simulink model "topology_comparison_cur"  (R2024b)
settings: Solver=ode23tb  StartTime=0.0  StopTime=0.15  MaxStep=1e-5  MinStep=1e-8  RelTol=1e-4
InitFcn:
  | sw_freq=60e3;
  | 
  | meas_delay=0.1;
  | 
  | V_high=80;
  | V_low=70;
  | 
  | L_ind=300e-6;
  | L_res=20e-3;
  | MOS_Ron=10e-3;
  | MOS_Vfw=1.2;
  | DIO_Vfw=1;
  | DIO_Ron=1e-3;
  | TRC_Res=5e-3;
  | 
  | buck_p=0.01;
  | buck_i=2;
  | 
  | inter_bdc_p=0.01;
  | inter_bdc_i=2;
  | 
  | asym_bdc_p=0.01;
  | asym_bdc_i=2;
values from neighbouring files (symbols this model uses):
  i_low_ref = 0.25    [compare_conv_curr.m]
  mode = 0    [compare_conv_curr.m]
libraries: spsGroundLib x33, spsSeriesRLCBranchLib x33, spsMosfetLib x18, spsDCVoltageSourceLib x14, spsMeanLib x10, slpidlib x10, spsMultimeterLib x6, spsVoltageMeasurementLib x4, spsDiodeLib x2, spsCurrentMeasurementLib x2, sps_lib x1
(part 1 of 2)
settings Model: SimulationMode=rapid-accelerator  Creator=adamo  LastModifiedBy=adamo
settings DebuggingCC: MaskedZcDiagnostic=none  IgnoredZcDiagnostic=none
settings HardwareCC: ProdHWDeviceType=AMD->x86-64 (Windows64)
settings RTWCC: BuildConfiguration=Faster Runs  CheckMdlBeforeBuild=Error
settings GRTTargetCC: OptimizeReductions=on
settings SimscapeCC: SimscapeCompileComponentReuse=on  SimscapeCompileArtifactsDiskCache=on

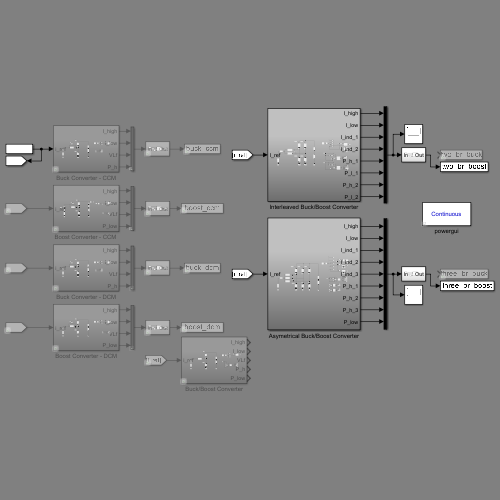
[thumbnail: Simulink's stored preview of the top-level diagram]
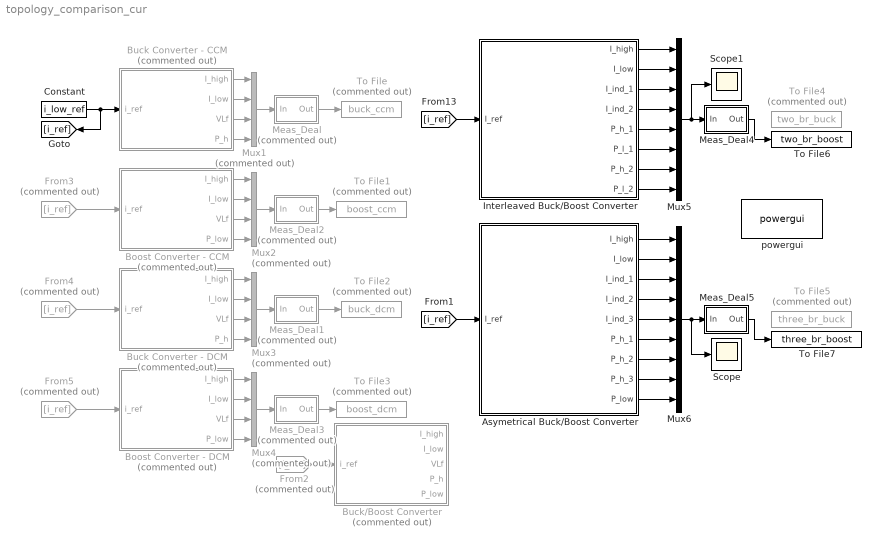
== system topology_comparison_cur ==
  Asymetrical Buck/Boost Converter : Subsystem
  "Boost Converter - CCM " : Subsystem  Commented=on
  Boost Converter - DCM : Subsystem  Commented=on
  Buck Converter - CCM : Subsystem  Commented=on
  Buck Converter - DCM : Subsystem  Commented=on
  Buck/Boost Converter : Subsystem  Commented=on
  Constant : Constant  Value=i_low_ref
  From{2..5} (4 alike) : From  Commented=on  GotoTag=i_ref
  Interleaved Buck/Boost Converter : Subsystem
  Meas_Deal : Subsystem  Commented=on
  Meas_Deal1 : Subsystem  Commented=on
  Meas_Deal2 : Subsystem  Commented=on
  Meas_Deal3 : Subsystem  Commented=on
  Meas_Deal4 : Subsystem
  Meas_Deal5 : Subsystem
  Mux{1..4} (4 alike) : Mux  Commented=on
  Mux5 : Mux  Inputs=8
  Mux6 : Mux  Inputs=9
  Scope : Scope
  Scope1 : Scope
  To File : ToFile  Commented=on  Filename=buck_ccm
  To File1 : ToFile  Commented=on  Filename=boost_ccm
  To File2 : ToFile  Commented=on  Filename=buck_dcm
  To File3 : ToFile  Commented=on  Filename=boost_dcm
  To File4 : ToFile  Commented=on  Filename=two_br_buck
  To File5 : ToFile  Commented=on  Filename=three_br_buck
  To File6 : ToFile  Filename=two_br_boost
  To File7 : ToFile  Filename=three_br_boost
  powergui : sps_lib/powergui  Priority=1  SimulationMode=Continuous  SampleTime=50e-6  frequency=60  Iterations=50  frequencyindice=0  Pbase=100e6  ErrMax=1e-4  UnitsV=kV  UnitsW=MW  buscounter=0  FunctionMessages=off  echomessages=off  EnableUseOfTLC=off  CurrentSourceSwitches=off  DisableSnubberDevices=on  DisableRonSwitches=off  DisableVfSwitches=off  DisplayEquations=off  AutomaticDiscreteSolvers=off  SolverType=Tustin/Backward Euler (TBE)  Interpol=off  ExternalGateDelay=off  methode=on  Ts=100  x0status=blocks  SPID=on  SwTol=0  HookPort=off  NonlinearTolerance=1e-4  nMaxIteration=100  ContinueOnMaxIteration=off  RestoreLinks=warning  ResistiveCurrentMeasurement=off  Frange=[0:2:500]  Ylog=off  Xlog=on  ShowGrid=off  save=off  variable=ZData  structure=0  ZoomFFT=off  StartTime=0.0  cycles=1  DisplayStyle=1  fundamental=60  FreqAxis=off  MaxFrequency=1000  frequencyindicesteady=1  RmsSteady=1  display=off
  wires:
  Buck Converter - CCM/2(I_low) -> Mux1/2
  Constant/1 -> [i_ref], Buck Converter - CCM/1(i_ref)
  [i_ref] -> Interleaved Buck/Boost Converter/1(I_ref)
  [i_ref] -> Asymetrical Buck/Boost Converter/1(I_ref)
  Buck Converter - CCM/3(VLf) -> Mux1/3
  Buck Converter - CCM/4(P_h) -> Mux1/4
  Meas_Deal/1(Out) -> To File/1
  From3/1 -> "Boost Converter - CCM "/1(i_ref)
  Meas_Deal2/1(Out) -> To File1/1
  "Boost Converter - CCM "/4(P_low) -> Mux2/4
  "Boost Converter - CCM "/3(VLf) -> Mux2/3
  "Boost Converter - CCM "/1(I_high) -> Mux2/1
  "Boost Converter - CCM "/2(I_low) -> Mux2/2
  Mux2/1 -> Meas_Deal2/1(In)
  From2/1 -> Buck/Boost Converter/1(i_ref)
  Buck Converter - CCM/1(I_high) -> Mux1/1
  Meas_Deal1/1(Out) -> To File2/1
  Meas_Deal3/1(Out) -> To File3/1
  Boost Converter - DCM/3(VLf) -> Mux4/3
  Buck Converter - DCM/3(VLf) -> Mux3/3
  Mux3/1 -> Meas_Deal1/1(In)
  Buck Converter - DCM/2(I_low) -> Mux3/2
  Buck Converter - DCM/4(P_h) -> Mux3/4
  Mux4/1 -> Meas_Deal3/1(In)
  From4/1 -> Buck Converter - DCM/1(i_ref)
  Boost Converter - DCM/2(I_low) -> Mux4/2
  Boost Converter - DCM/4(P_low) -> Mux4/4
  Buck Converter - DCM/1(I_high) -> Mux3/1
  From5/1 -> Boost Converter - DCM/1(i_ref)
  Boost Converter - DCM/1(I_high) -> Mux4/1
  Mux1/1 -> Meas_Deal/1(In)
  Interleaved Buck/Boost Converter/1(I_high) -> Mux5/1
  Interleaved Buck/Boost Converter/2(I_low) -> Mux5/2
  Interleaved Buck/Boost Converter/3(I_ind_1) -> Mux5/3
  Interleaved Buck/Boost Converter/4(I_ind_2) -> Mux5/4
  Interleaved Buck/Boost Converter/5(P_h_1) -> Mux5/5
  Interleaved Buck/Boost Converter/6(P_l_1) -> Mux5/6
  Interleaved Buck/Boost Converter/7(P_h_2) -> Mux5/7
  Interleaved Buck/Boost Converter/8(P_l_2) -> Mux5/8
  Meas_Deal4/1(Out) -> To File6/1
  Mux5/1 -> Scope1/1, Meas_Deal4/1(In)
  Asymetrical Buck/Boost Converter/1(I_high) -> Mux6/1
  Asymetrical Buck/Boost Converter/2(I_low) -> Mux6/2
  Asymetrical Buck/Boost Converter/3(I_ind_1) -> Mux6/3
  Asymetrical Buck/Boost Converter/4(I_ind_2) -> Mux6/4
  Asymetrical Buck/Boost Converter/5(I_ind_3) -> Mux6/5
  Asymetrical Buck/Boost Converter/6(P_h_1) -> Mux6/6
  Asymetrical Buck/Boost Converter/7(P_h_2) -> Mux6/7
  Asymetrical Buck/Boost Converter/8(P_h_3) -> Mux6/8
  Asymetrical Buck/Boost Converter/9(P_low) -> Mux6/9
  Mux6/1 -> Scope/1, Meas_Deal5/1(In)
  Meas_Deal5/1(Out) -> To File7/1

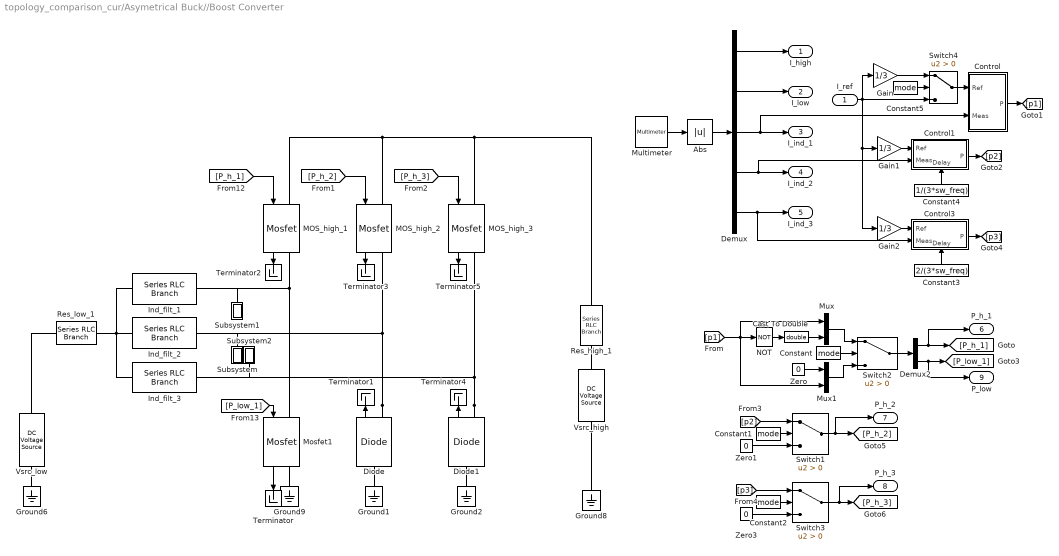
== system topology_comparison_cur/Asymetrical Buck//Boost Converter ==
  I_ref : Inport
  Abs : Abs  SaturateOnIntegerOverflow=off
  Cast To Double : DataTypeConversion  OutDataTypeStr=double  SaturateOnIntegerOverflow=off  RndMeth=Floor
  Constant{,1..2,5} (4 alike) : Constant  Value=mode
  Constant3 : Constant  Value=2/(3*sw_freq)
  Constant4 : Constant  Value=1/(3*sw_freq)
  Control : Subsystem
  Control1 : Subsystem
      settings: PortSchema="{\"entries\":[{\"content\":{\"sides\":[{\"content\":{\"connectorIds\":[\"In1\",\"In2\"]},\"type\":\"ConnectorPlacement.EquallySpacedRectSide\",\"uuid\":\"44975c06-6cb3-4b92-aa2e-c11b859d13e4\"},{\"content\":{\"connectorIds\":[\"Out1\"],\"side\":\"RIGHT\"},\"type\":\"ConnectorPlacement.EquallySpacedRectSide\",\"uuid\":\"ebdc9065-5b19-4aa7-8841-916fd82a5d31\"},{\"content\":{\"side\":\"TOP\"},\"type\":\"ConnectorPlacement.EquallySpacedRectSide\",\"uuid\":\"027925ea-888b-4bcf-b8a4-44694d0e275e\"},{\"content\":{\"connectorIds\":[\"In3\"],\"side\":\"BOTTOM\"},\"type\":\"ConnectorPlacement.EquallySpacedRectSide\",\"uuid\":\"415fb0af-dd9a-4309-9118-76332ed11379\"}]},\"type\":\"ConnectorPlacement.EquallySpacedConnector\",\"uuid\":\"3cd19595-535e-42c3-a0e6-40045bedee28\"}],\"packageUris\":[\"http://schema.mathworks.com/mf0/Connector/R2020b\"],\"version\":\"1.0\"}"
  Control3 : Subsystem
      settings: PortSchema="{\"entries\":[{\"content\":{\"sides\":[{\"content\":{\"connectorIds\":[\"In1\",\"In2\"]},\"type\":\"ConnectorPlacement.EquallySpacedRectSide\",\"uuid\":\"44975c06-6cb3-4b92-aa2e-c11b859d13e4\"},{\"content\":{\"connectorIds\":[\"Out1\"],\"side\":\"RIGHT\"},\"type\":\"ConnectorPlacement.EquallySpacedRectSide\",\"uuid\":\"ebdc9065-5b19-4aa7-8841-916fd82a5d31\"},{\"content\":{\"side\":\"TOP\"},\"type\":\"ConnectorPlacement.EquallySpacedRectSide\",\"uuid\":\"027925ea-888b-4bcf-b8a4-44694d0e275e\"},{\"content\":{\"connectorIds\":[\"In3\"],\"side\":\"BOTTOM\"},\"type\":\"ConnectorPlacement.EquallySpacedRectSide\",\"uuid\":\"9488b47a-c58c-42e9-bacd-7bb9f563b775\"}]},\"type\":\"ConnectorPlacement.EquallySpacedConnector\",\"uuid\":\"3cd19595-535e-42c3-a0e6-40045bedee28\"}],\"packageUris\":[\"http://schema.mathworks.com/mf0/Connector/R2020b\"],\"version\":\"1.0\"}"
  Demux : Demux  Outputs=5
  Demux2 : Demux  Outputs=2
  Diode : spsDiodeLib/Diode  Ron=0.001  Lon=0  Vf=0.8  IC=0  UseSnubber=0  Rs=500  Cs=250e-9  Measurements=on
  Diode1 : spsDiodeLib/Diode  Ron=0.001  Lon=0  Vf=0.8  IC=0  UseSnubber=0  Rs=500  Cs=250e-9  Measurements=on
  Gain : Gain  Gain=1/3
  Gain1 : Gain  Gain=1/3
  Gain2 : Gain  Gain=1/3
  Ground{1..2,6,8..9} (5 alike) : spsGroundLib/Ground  LConnTagsString=a
  Ind_filt_1 : spsSeriesRLCBranchLib/Series RLC Branch  LConnTagsString=__new0  RConnTagsString=__new0  BranchType=RL  Resistance=L_res  Inductance=L_ind*7  SetiL0=off  InitialCurrent=10  Capacitance=1e-6  Setx0=off  InitialVoltage=0  Measurements=Branch current
  Ind_filt_2 : spsSeriesRLCBranchLib/Series RLC Branch  LConnTagsString=__new0  RConnTagsString=__new0  BranchType=RL  Resistance=L_res  Inductance=L_ind*7  SetiL0=off  InitialCurrent=10  Capacitance=1e-6  Setx0=off  InitialVoltage=0  Measurements=Branch current
  Ind_filt_3 : spsSeriesRLCBranchLib/Series RLC Branch  LConnTagsString=__new0  RConnTagsString=__new0  BranchType=RL  Resistance=L_res  Inductance=L_ind*7  SetiL0=off  InitialCurrent=10  Capacitance=1e-6  Setx0=off  InitialVoltage=0  Measurements=Branch current
  MOS_high_1 : spsMosfetLib/Mosfet  Ron=MOS_Ron  Lon=0  Rd=DIO_Ron  Vfd=MOS_Vfw  IC=0  Rs=1e5  Cs=inf  Measurements=on
  MOS_high_2 : spsMosfetLib/Mosfet  Ron=MOS_Ron  Lon=0  Rd=DIO_Ron  Vfd=MOS_Vfw  IC=0  Rs=1e5  Cs=inf  Measurements=on
  MOS_high_3 : spsMosfetLib/Mosfet  Ron=MOS_Ron  Lon=0  Rd=DIO_Ron  Vfd=MOS_Vfw  IC=0  Rs=1e5  Cs=inf  Measurements=on
  Mosfet1 : spsMosfetLib/Mosfet  Ron=0.1  Lon=0  Rd=0.01  Vfd=0  IC=0  Rs=1e5  Cs=inf  Measurements=on
  Multimeter : spsMultimeterLib/Multimeter  L=9  sel=[4 5 1 2 3]  yselected={}  Gain=[1 1 1 1 1]  OutputType=Complex  PlotAtSimulationStop=off  PhasorSimulation=off
  Mux : Mux  Inputs=2
  Mux1 : Mux  Inputs=2
  NOT : Logic  Operator=NOT  IconShape=distinctive  AllPortsSameDT=off  OutDataTypeStr=boolean
  Res_high_1 : spsSeriesRLCBranchLib/Series RLC Branch  LConnTagsString=__new0  RConnTagsString=__new0  BranchType=R  Resistance=TRC_Res  Inductance=1e-3  SetiL0=off  InitialCurrent=0  Capacitance=1e-6  Setx0=off  InitialVoltage=0  Measurements=Branch current
  Res_low_1 : spsSeriesRLCBranchLib/Series RLC Branch  LConnTagsString=__new0  RConnTagsString=__new0  BranchType=R  Resistance=TRC_Res  Inductance=1e-3  SetiL0=off  InitialCurrent=0  Capacitance=1e-6  Setx0=off  InitialVoltage=0  Measurements=Branch current
  Subsystem : Subsystem
      settings: PortSchema="{\"entries\":[{\"content\":{\"sides\":[{\"content\":{},\"type\":\"ConnectorPlacement.EquallySpacedRectSide\",\"uuid\":\"333a472d-5660-403e-9749-9e5a485a4e51\"},{\"content\":{\"side\":\"RIGHT\"},\"type\":\"ConnectorPlacement.EquallySpacedRectSide\",\"uuid\":\"46e3a3df-9b43-4056-bf49-6d97e0ff375e\"},{\"content\":{\"connectorIds\":[\"LConn1\"],\"side\":\"TOP\"},\"type\":\"ConnectorPlacement.EquallySpacedRectSide\",\"uuid\":\"a9be43b9-3284-437d-b483-2a714199e3a2\"}]},\"type\":\"ConnectorPlacement.EquallySpacedConnector\",\"uuid\":\"6030dd83-63ea-4a67-9f73-95d000b3af89\"}],\"packageUris\":[\"http://schema.mathworks.com/mf0/Connector/R2020b\"],\"version\":\"1.0\"}"
  Subsystem1 : Subsystem
      settings: PortSchema="{\"entries\":[{\"content\":{\"sides\":[{\"content\":{},\"type\":\"ConnectorPlacement.EquallySpacedRectSide\",\"uuid\":\"333a472d-5660-403e-9749-9e5a485a4e51\"},{\"content\":{\"side\":\"RIGHT\"},\"type\":\"ConnectorPlacement.EquallySpacedRectSide\",\"uuid\":\"46e3a3df-9b43-4056-bf49-6d97e0ff375e\"},{\"content\":{\"connectorIds\":[\"LConn1\"],\"side\":\"TOP\"},\"type\":\"ConnectorPlacement.EquallySpacedRectSide\",\"uuid\":\"a9be43b9-3284-437d-b483-2a714199e3a2\"}]},\"type\":\"ConnectorPlacement.EquallySpacedConnector\",\"uuid\":\"6030dd83-63ea-4a67-9f73-95d000b3af89\"}],\"packageUris\":[\"http://schema.mathworks.com/mf0/Connector/R2020b\"],\"version\":\"1.0\"}"
  Subsystem2 : Subsystem
      settings: PortSchema="{\"entries\":[{\"content\":{\"sides\":[{\"content\":{},\"type\":\"ConnectorPlacement.EquallySpacedRectSide\",\"uuid\":\"333a472d-5660-403e-9749-9e5a485a4e51\"},{\"content\":{\"side\":\"RIGHT\"},\"type\":\"ConnectorPlacement.EquallySpacedRectSide\",\"uuid\":\"46e3a3df-9b43-4056-bf49-6d97e0ff375e\"},{\"content\":{\"connectorIds\":[\"LConn1\"],\"side\":\"TOP\"},\"type\":\"ConnectorPlacement.EquallySpacedRectSide\",\"uuid\":\"a9be43b9-3284-437d-b483-2a714199e3a2\"}]},\"type\":\"ConnectorPlacement.EquallySpacedConnector\",\"uuid\":\"6030dd83-63ea-4a67-9f73-95d000b3af89\"}],\"packageUris\":[\"http://schema.mathworks.com/mf0/Connector/R2020b\"],\"version\":\"1.0\"}"
  Switch{1..4} (4 alike) : Switch  Criteria=u2 > Threshold  SaturateOnIntegerOverflow=off  InputSameDT=off
  Terminator{,1..5} (6 alike) : Terminator
  Vsrc_high : spsDCVoltageSourceLib/DC Voltage Source  Amplitude=V_high  Measurements=None
  Vsrc_low : spsDCVoltageSourceLib/DC Voltage Source  Amplitude=V_low  Measurements=None
  Zero : Constant  Value=0  OutDataTypeStr=Inherit: Inherit via back propagation
  Zero1 : Constant  Value=0  OutDataTypeStr=Inherit: Inherit via back propagation
  Zero3 : Constant  Value=0  OutDataTypeStr=Inherit: Inherit via back propagation
  I_high : Outport
  I_low : Outport  Port=2
  I_ind_1 : Outport  Port=3
  I_ind_2 : Outport  Port=4
  I_ind_3 : Outport  Port=5
  P_h_1 : Outport  Port=6
  P_h_2 : Outport  Port=7
  P_h_3 : Outport  Port=8
  P_low : Outport  Port=9
  wires:
  [P_h_1] -> MOS_high_1/1
  MOS_high_1/1 -> Terminator2/1
  Mosfet1/1 -> Terminator/1
  [P_low_1] -> Mosfet1/1
  Diode/1 -> Terminator1/1
  MOS_high_2/1 -> Terminator3/1
  Diode1/1 -> Terminator4/1
  MOS_high_3/1 -> Terminator5/1
  [P_h_3] -> MOS_high_3/1
  Multimeter/1 -> Abs/1
  Switch2/1 -> Demux2/1
  Mux/1 -> Switch2/1
  Demux2/2 -> P_low/1, [P_low_1]
  Demux2/1 -> P_h_1/1, [P_h_1]
  Constant/1 -> Switch2/2
  I_ref/1 -> Gain/1, Switch4/3, Gain2/1, Gain1/1
  [P_h_2] -> MOS_high_2/1
  Demux/5 -> Control3/2(Meas), I_ind_3/1
  Demux/3 -> Control/2(Meas), I_ind_1/1
  Mux1/1 -> Switch2/3
  Cast To Double/1 -> Mux/2
  Demux/2 -> I_low/1
  Demux/1 -> I_high/1
  Abs/1 -> Demux/1
  Switch4/1 -> Control/1(Ref)
  Control/1(P) -> [p1]
  Control1/1(P) -> [p2]
  Gain1/1 -> Control1/1(Ref)
  Demux/4 -> Control1/2(Meas), I_ind_2/1
  Gain2/1 -> Control3/1(Ref)
  Control3/1(P) -> [p3]
  Switch3/1 -> P_h_3/1, [P_h_3]
  Switch1/1 -> P_h_2/1, [P_h_2]
  Constant1/1 -> Switch1/2
  [p2] -> Switch1/1
  Zero1/1 -> Switch1/3
  Constant2/1 -> Switch3/2
  [p3] -> Switch3/1
  Zero3/1 -> Switch3/3
  Constant4/1 -> Control1/3(Delay)
  Constant3/1 -> Control3/3(Delay)
  NOT/1 -> Cast To Double/1
  [p1] -> NOT/1, Mux/1, Mux1/2
  Constant5/1 -> Switch4/2
  Gain/1 -> Switch4/1
  Zero/1 -> Mux1/1
  connections:
  Diode/RConn1 -- Ind_filt_2/LConn1 -- Subsystem/LConn1 -- MOS_high_2/RConn1
  MOS_high_1/RConn1 -- Ind_filt_1/LConn1 -- Subsystem1/LConn1 -- Mosfet1/LConn1
  Ground8/LConn1 -- Vsrc_high/LConn1
  Mosfet1/RConn1 -- Ground9/LConn1
  Ground6/LConn1 -- Vsrc_low/LConn1
  Diode/LConn1 -- Ground1/LConn1
  Diode1/RConn1 -- Ind_filt_3/LConn1 -- Subsystem2/LConn1 -- MOS_high_3/RConn1
  Diode1/LConn1 -- Ground2/LConn1
  Res_low_1/RConn1 -- Vsrc_low/RConn1
  Res_high_1/LConn1 -- Vsrc_high/RConn1
  Ind_filt_2/RConn1 -- Res_low_1/LConn1 -- Ind_filt_3/RConn1 -- Ind_filt_1/RConn1
  Res_high_1/RConn1 -- MOS_high_1/LConn1 -- MOS_high_2/LConn1 -- MOS_high_3/LConn1

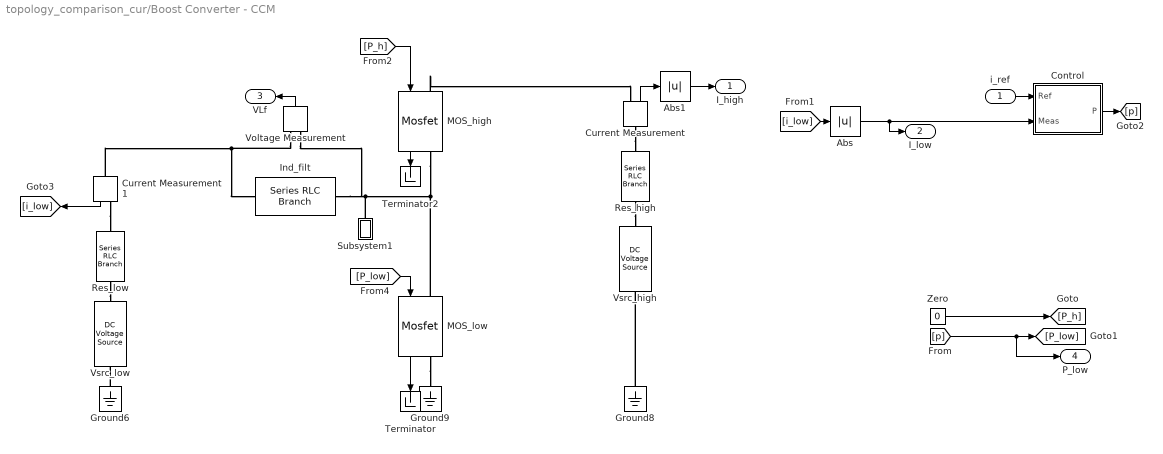
== system topology_comparison_cur/Boost Converter - CCM  ==
  i_ref : Inport
  Abs : Abs  SaturateOnIntegerOverflow=off
  Abs1 : Abs  SaturateOnIntegerOverflow=off
  Control : Subsystem
  Current Measurement : spsCurrentMeasurementLib/Current Measurement  PhasorSimulation=off  OutputType=Complex  PSBequivalent=0
  Current Measurement1 : spsCurrentMeasurementLib/Current Measurement  PhasorSimulation=off  OutputType=Complex  PSBequivalent=0
  Ground6 : spsGroundLib/Ground  LConnTagsString=a
  Ground8 : spsGroundLib/Ground  LConnTagsString=a
  Ground9 : spsGroundLib/Ground  LConnTagsString=a
  Ind_filt : spsSeriesRLCBranchLib/Series RLC Branch  LConnTagsString=__new0  RConnTagsString=__new0  BranchType=RL  Resistance=L_res  Inductance=L_ind  SetiL0=off  InitialCurrent=20  Capacitance=1e-6  Setx0=off  InitialVoltage=0  Measurements=None
  MOS_high : spsMosfetLib/Mosfet  Ron=MOS_Ron  Lon=0  Rd=DIO_Ron  Vfd=MOS_Vfw  IC=0  Rs=1e5  Cs=inf  Measurements=on
  MOS_low : spsMosfetLib/Mosfet  Ron=MOS_Ron  Lon=0  Rd=DIO_Ron  Vfd=MOS_Vfw  IC=0  Rs=1e5  Cs=inf  Measurements=on
  Res_high : spsSeriesRLCBranchLib/Series RLC Branch  LConnTagsString=__new0  RConnTagsString=__new0  BranchType=R  Resistance=TRC_Res  Inductance=1e-3  SetiL0=off  InitialCurrent=0  Capacitance=1e-6  Setx0=off  InitialVoltage=0  Measurements=None
  Res_low : spsSeriesRLCBranchLib/Series RLC Branch  LConnTagsString=__new0  RConnTagsString=__new0  BranchType=R  Resistance=TRC_Res  Inductance=1e-3  SetiL0=off  InitialCurrent=0  Capacitance=1e-6  Setx0=off  InitialVoltage=0  Measurements=None
  Subsystem1 : Subsystem
      settings: PortSchema="{\"entries\":[{\"content\":{\"sides\":[{\"content\":{},\"type\":\"ConnectorPlacement.EquallySpacedRectSide\",\"uuid\":\"333a472d-5660-403e-9749-9e5a485a4e51\"},{\"content\":{\"side\":\"RIGHT\"},\"type\":\"ConnectorPlacement.EquallySpacedRectSide\",\"uuid\":\"46e3a3df-9b43-4056-bf49-6d97e0ff375e\"},{\"content\":{\"connectorIds\":[\"LConn1\"],\"side\":\"TOP\"},\"type\":\"ConnectorPlacement.EquallySpacedRectSide\",\"uuid\":\"a9be43b9-3284-437d-b483-2a714199e3a2\"}]},\"type\":\"ConnectorPlacement.EquallySpacedConnector\",\"uuid\":\"6030dd83-63ea-4a67-9f73-95d000b3af89\"}],\"packageUris\":[\"http://schema.mathworks.com/mf0/Connector/R2020b\"],\"version\":\"1.0\"}"
  Terminator : Terminator
  Terminator2 : Terminator
  Voltage Measurement : spsVoltageMeasurementLib/Voltage Measurement  PhasorSimulation=off  OutputType=Complex  PSBequivalent=0
  Vsrc_high : spsDCVoltageSourceLib/DC Voltage Source  Amplitude=V_high  Measurements=None
  Vsrc_low : spsDCVoltageSourceLib/DC Voltage Source  Amplitude=V_low  Measurements=None
  Zero : Constant  Value=0  OutDataTypeStr=Inherit: Inherit via back propagation
  I_high : Outport
  I_low : Outport  Port=2
  VLf : Outport  Port=3
  P_low : Outport  Port=4
  wires:
  MOS_low/1 -> Terminator/1
  MOS_high/1 -> Terminator2/1
  [P_h] -> MOS_high/1
  [P_low] -> MOS_low/1
  Abs/1 -> I_low/1, Control/2(Meas)
  Zero/1 -> [P_h]
  i_ref/1 -> Control/1(Ref)
  [p] -> P_low/1, [P_low]
  Control/1(P) -> [p]
  Voltage Measurement/1 -> VLf/1
  Current Measurement/1 -> Abs1/1
  Current Measurement1/1 -> [i_low]
  [i_low] -> Abs/1
  Abs1/1 -> I_high/1
  connections:
  MOS_high/LConn1 -- Current Measurement/RConn1
  MOS_low/RConn1 -- Ground9/LConn1
  MOS_high/RConn1 -- Subsystem1/LConn1 -- Voltage Measurement/LConn1 -- Ind_filt/LConn1 -- MOS_low/LConn1
  Ground8/LConn1 -- Vsrc_high/LConn1
  Ground6/LConn1 -- Vsrc_low/LConn1
  Voltage Measurement/LConn2 -- Ind_filt/RConn1 -- Current Measurement1/LConn1
  Res_high/LConn1 -- Vsrc_high/RConn1
  Res_low/RConn1 -- Vsrc_low/RConn1
  Current Measurement/LConn1 -- Res_high/RConn1
  Current Measurement1/RConn1 -- Res_low/LConn1

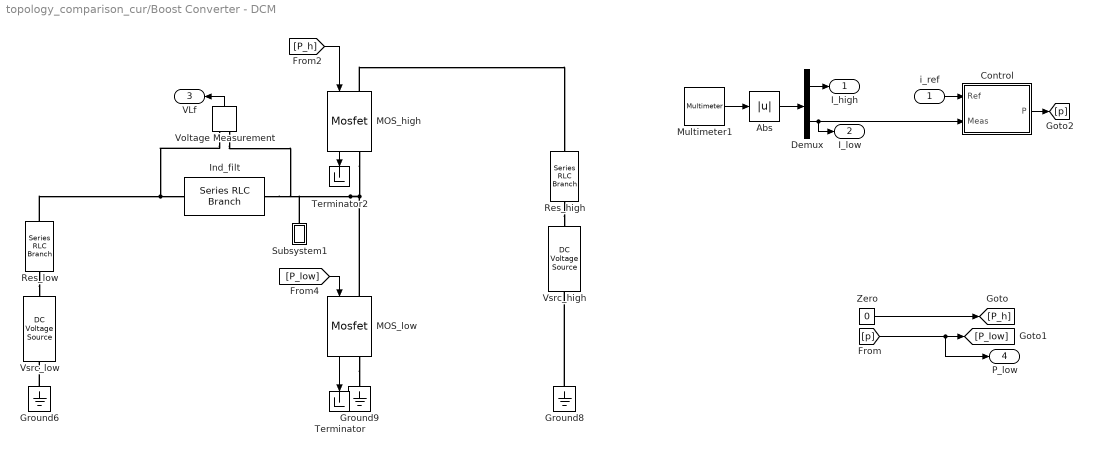
== system topology_comparison_cur/Boost Converter - DCM ==
  i_ref : Inport
  Abs : Abs  SaturateOnIntegerOverflow=off
  Control : Subsystem
  Demux : Demux  Outputs=2
  Ground6 : spsGroundLib/Ground  LConnTagsString=a
  Ground8 : spsGroundLib/Ground  LConnTagsString=a
  Ground9 : spsGroundLib/Ground  LConnTagsString=a
  Ind_filt : spsSeriesRLCBranchLib/Series RLC Branch  LConnTagsString=__new0  RConnTagsString=__new0  BranchType=RL  Resistance=L_res  Inductance=L_ind/30  SetiL0=off  InitialCurrent=20  Capacitance=1e-6  Setx0=off  InitialVoltage=0  Measurements=None
  MOS_high : spsMosfetLib/Mosfet  Ron=MOS_Ron  Lon=0  Rd=DIO_Ron  Vfd=MOS_Vfw  IC=0  Rs=1e5  Cs=inf  Measurements=on
  MOS_low : spsMosfetLib/Mosfet  Ron=MOS_Ron  Lon=0  Rd=DIO_Ron  Vfd=MOS_Vfw  IC=0  Rs=1e5  Cs=inf  Measurements=on
  Multimeter1 : spsMultimeterLib/Multimeter  L=6  sel=[1 2]  yselected={}  Gain=[1 1]  OutputType=Complex  PlotAtSimulationStop=off  PhasorSimulation=off
  Res_high : spsSeriesRLCBranchLib/Series RLC Branch  LConnTagsString=__new0  RConnTagsString=__new0  BranchType=R  Resistance=TRC_Res  Inductance=1e-3  SetiL0=off  InitialCurrent=0  Capacitance=1e-6  Setx0=off  InitialVoltage=0  Measurements=Branch current
  Res_low : spsSeriesRLCBranchLib/Series RLC Branch  LConnTagsString=__new0  RConnTagsString=__new0  BranchType=R  Resistance=TRC_Res  Inductance=1e-3  SetiL0=off  InitialCurrent=0  Capacitance=1e-6  Setx0=off  InitialVoltage=0  Measurements=Branch current
  Subsystem1 : Subsystem
      settings: PortSchema="{\"entries\":[{\"content\":{\"sides\":[{\"content\":{},\"type\":\"ConnectorPlacement.EquallySpacedRectSide\",\"uuid\":\"333a472d-5660-403e-9749-9e5a485a4e51\"},{\"content\":{\"side\":\"RIGHT\"},\"type\":\"ConnectorPlacement.EquallySpacedRectSide\",\"uuid\":\"46e3a3df-9b43-4056-bf49-6d97e0ff375e\"},{\"content\":{\"connectorIds\":[\"LConn1\"],\"side\":\"TOP\"},\"type\":\"ConnectorPlacement.EquallySpacedRectSide\",\"uuid\":\"a9be43b9-3284-437d-b483-2a714199e3a2\"}]},\"type\":\"ConnectorPlacement.EquallySpacedConnector\",\"uuid\":\"6030dd83-63ea-4a67-9f73-95d000b3af89\"}],\"packageUris\":[\"http://schema.mathworks.com/mf0/Connector/R2020b\"],\"version\":\"1.0\"}"
  Terminator : Terminator
  Terminator2 : Terminator
  Voltage Measurement : spsVoltageMeasurementLib/Voltage Measurement  PhasorSimulation=off  OutputType=Complex  PSBequivalent=0
  Vsrc_high : spsDCVoltageSourceLib/DC Voltage Source  Amplitude=V_high  Measurements=None
  Vsrc_low : spsDCVoltageSourceLib/DC Voltage Source  Amplitude=V_low  Measurements=None
  Zero : Constant  Value=0  OutDataTypeStr=Inherit: Inherit via back propagation
  I_high : Outport
  I_low : Outport  Port=2
  VLf : Outport  Port=3
  P_low : Outport  Port=4
  wires:
  MOS_low/1 -> Terminator/1
  MOS_high/1 -> Terminator2/1
  [P_h] -> MOS_high/1
  [P_low] -> MOS_low/1
  Demux/1 -> I_high/1
  Demux/2 -> I_low/1, Control/2(Meas)
  Zero/1 -> [P_h]
  i_ref/1 -> Control/1(Ref)
  Multimeter1/1 -> Abs/1
  [p] -> P_low/1, [P_low]
  Abs/1 -> Demux/1
  Control/1(P) -> [p]
  Voltage Measurement/1 -> VLf/1
  connections:
  MOS_high/LConn1 -- Res_high/RConn1
  MOS_low/RConn1 -- Ground9/LConn1
  MOS_high/RConn1 -- MOS_low/LConn1 -- Voltage Measurement/LConn1 -- Ind_filt/LConn1 -- Subsystem1/LConn1
  Ground8/LConn1 -- Vsrc_high/LConn1
  Ground6/LConn1 -- Vsrc_low/LConn1
  Res_low/LConn1 -- Ind_filt/RConn1 -- Voltage Measurement/LConn2
  Res_high/LConn1 -- Vsrc_high/RConn1
  Res_low/RConn1 -- Vsrc_low/RConn1

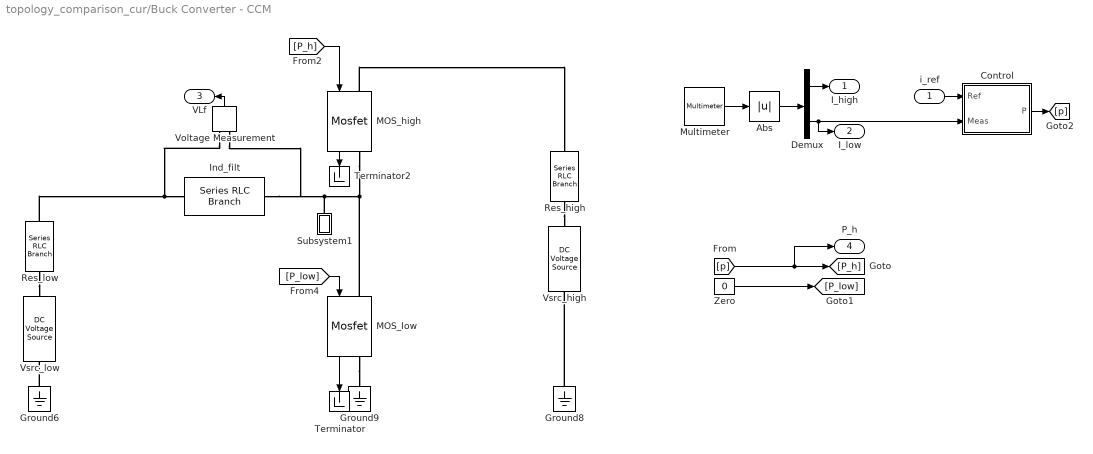
== system topology_comparison_cur/Buck Converter - CCM ==
  i_ref : Inport
  Abs : Abs  SaturateOnIntegerOverflow=off
  Control : Subsystem
  Demux : Demux  Outputs=2
  Ground6 : spsGroundLib/Ground  LConnTagsString=a
  Ground8 : spsGroundLib/Ground  LConnTagsString=a
  Ground9 : spsGroundLib/Ground  LConnTagsString=a
  Ind_filt : spsSeriesRLCBranchLib/Series RLC Branch  LConnTagsString=__new0  RConnTagsString=__new0  BranchType=RL  Resistance=L_res  Inductance=L_ind  SetiL0=off  InitialCurrent=20  Capacitance=1e-6  Setx0=off  InitialVoltage=0  Measurements=None
  MOS_high : spsMosfetLib/Mosfet  Ron=MOS_Ron  Lon=0  Rd=DIO_Ron  Vfd=MOS_Vfw  IC=0  Rs=1e5  Cs=inf  Measurements=on
  MOS_low : spsMosfetLib/Mosfet  Ron=MOS_Ron  Lon=0  Rd=DIO_Ron  Vfd=MOS_Vfw  IC=0  Rs=1e5  Cs=inf  Measurements=on
  Multimeter : spsMultimeterLib/Multimeter  L=6  sel=[3 4]  yselected={}  Gain=[1 1]  OutputType=Complex  PlotAtSimulationStop=off  PhasorSimulation=off
  Res_high : spsSeriesRLCBranchLib/Series RLC Branch  LConnTagsString=__new0  RConnTagsString=__new0  BranchType=R  Resistance=TRC_Res  Inductance=1e-3  SetiL0=off  InitialCurrent=0  Capacitance=1e-6  Setx0=off  InitialVoltage=0  Measurements=Branch current
  Res_low : spsSeriesRLCBranchLib/Series RLC Branch  LConnTagsString=__new0  RConnTagsString=__new0  BranchType=R  Resistance=TRC_Res  Inductance=1e-3  SetiL0=off  InitialCurrent=0  Capacitance=1e-6  Setx0=off  InitialVoltage=0  Measurements=Branch current
  Subsystem1 : Subsystem
      settings: PortSchema="{\"entries\":[{\"content\":{\"sides\":[{\"content\":{},\"type\":\"ConnectorPlacement.EquallySpacedRectSide\",\"uuid\":\"333a472d-5660-403e-9749-9e5a485a4e51\"},{\"content\":{\"side\":\"RIGHT\"},\"type\":\"ConnectorPlacement.EquallySpacedRectSide\",\"uuid\":\"46e3a3df-9b43-4056-bf49-6d97e0ff375e\"},{\"content\":{\"connectorIds\":[\"LConn1\"],\"side\":\"TOP\"},\"type\":\"ConnectorPlacement.EquallySpacedRectSide\",\"uuid\":\"a9be43b9-3284-437d-b483-2a714199e3a2\"}]},\"type\":\"ConnectorPlacement.EquallySpacedConnector\",\"uuid\":\"6030dd83-63ea-4a67-9f73-95d000b3af89\"}],\"packageUris\":[\"http://schema.mathworks.com/mf0/Connector/R2020b\"],\"version\":\"1.0\"}"
  Terminator : Terminator
  Terminator2 : Terminator
  Voltage Measurement : spsVoltageMeasurementLib/Voltage Measurement  PhasorSimulation=off  OutputType=Complex  PSBequivalent=0
  Vsrc_high : spsDCVoltageSourceLib/DC Voltage Source  Amplitude=V_high  Measurements=None
  Vsrc_low : spsDCVoltageSourceLib/DC Voltage Source  Amplitude=V_low  Measurements=None
  Zero : Constant  Value=0  OutDataTypeStr=Inherit: Inherit via back propagation
  I_high : Outport
  I_low : Outport  Port=2
  VLf : Outport  Port=3
  P_h : Outport  Port=4
  wires:
  MOS_low/1 -> Terminator/1
  MOS_high/1 -> Terminator2/1
  [P_h] -> MOS_high/1
  [P_low] -> MOS_low/1
  Demux/1 -> I_high/1
  Demux/2 -> I_low/1, Control/2(Meas)
  [p] -> P_h/1, [P_h]
  i_ref/1 -> Control/1(Ref)
  Multimeter/1 -> Abs/1
  Zero/1 -> [P_low]
  Abs/1 -> Demux/1
  Control/1(P) -> [p]
  Voltage Measurement/1 -> VLf/1
  connections:
  MOS_high/LConn1 -- Res_high/RConn1
  MOS_low/RConn1 -- Ground9/LConn1
  MOS_high/RConn1 -- Subsystem1/LConn1 -- Voltage Measurement/LConn1 -- Ind_filt/LConn1 -- MOS_low/LConn1
  Ground8/LConn1 -- Vsrc_high/LConn1
  Ground6/LConn1 -- Vsrc_low/LConn1
  Res_low/LConn1 -- Voltage Measurement/LConn2 -- Ind_filt/RConn1
  Res_high/LConn1 -- Vsrc_high/RConn1
  Res_low/RConn1 -- Vsrc_low/RConn1

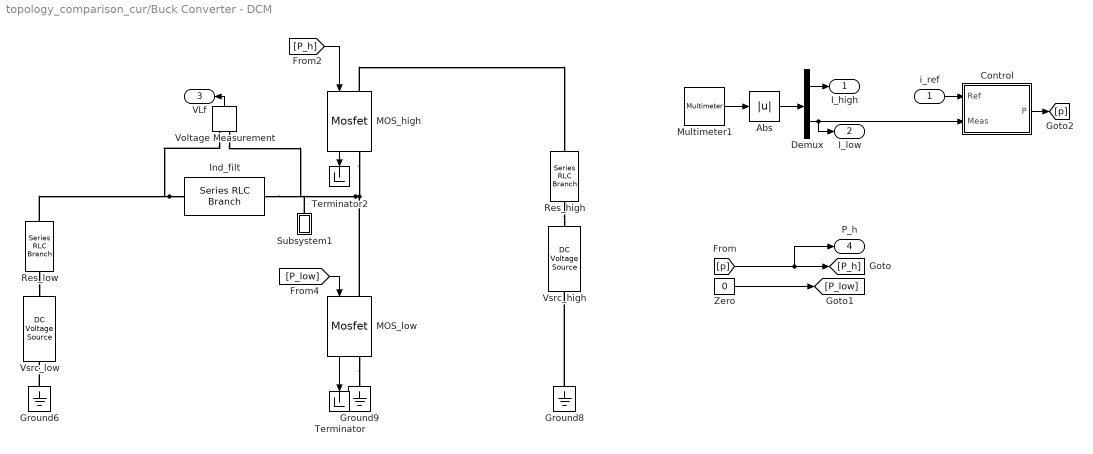
== system topology_comparison_cur/Buck Converter - DCM ==
  i_ref : Inport
  Abs : Abs  SaturateOnIntegerOverflow=off
  Control : Subsystem
  Demux : Demux  Outputs=2
  Ground6 : spsGroundLib/Ground  LConnTagsString=a
  Ground8 : spsGroundLib/Ground  LConnTagsString=a
  Ground9 : spsGroundLib/Ground  LConnTagsString=a
  Ind_filt : spsSeriesRLCBranchLib/Series RLC Branch  LConnTagsString=__new0  RConnTagsString=__new0  BranchType=RL  Resistance=L_res  Inductance=L_ind/30  SetiL0=off  InitialCurrent=20  Capacitance=1e-6  Setx0=off  InitialVoltage=0  Measurements=None
  MOS_high : spsMosfetLib/Mosfet  Ron=MOS_Ron  Lon=0  Rd=DIO_Ron  Vfd=MOS_Vfw  IC=0  Rs=1e5  Cs=inf  Measurements=on
  MOS_low : spsMosfetLib/Mosfet  Ron=MOS_Ron  Lon=0  Rd=DIO_Ron  Vfd=MOS_Vfw  IC=0  Rs=1e5  Cs=inf  Measurements=on
  Multimeter1 : spsMultimeterLib/Multimeter  L=6  sel=[5 6]  yselected={}  Gain=[1 1]  OutputType=Complex  PlotAtSimulationStop=off  PhasorSimulation=off
  Res_high : spsSeriesRLCBranchLib/Series RLC Branch  LConnTagsString=__new0  RConnTagsString=__new0  BranchType=R  Resistance=TRC_Res  Inductance=1e-3  SetiL0=off  InitialCurrent=0  Capacitance=1e-6  Setx0=off  InitialVoltage=0  Measurements=Branch current
  Res_low : spsSeriesRLCBranchLib/Series RLC Branch  LConnTagsString=__new0  RConnTagsString=__new0  BranchType=R  Resistance=TRC_Res  Inductance=1e-3  SetiL0=off  InitialCurrent=0  Capacitance=1e-6  Setx0=off  InitialVoltage=0  Measurements=Branch current
  Subsystem1 : Subsystem
      settings: PortSchema="{\"entries\":[{\"content\":{\"sides\":[{\"content\":{},\"type\":\"ConnectorPlacement.EquallySpacedRectSide\",\"uuid\":\"333a472d-5660-403e-9749-9e5a485a4e51\"},{\"content\":{\"side\":\"RIGHT\"},\"type\":\"ConnectorPlacement.EquallySpacedRectSide\",\"uuid\":\"46e3a3df-9b43-4056-bf49-6d97e0ff375e\"},{\"content\":{\"connectorIds\":[\"LConn1\"],\"side\":\"TOP\"},\"type\":\"ConnectorPlacement.EquallySpacedRectSide\",\"uuid\":\"a9be43b9-3284-437d-b483-2a714199e3a2\"}]},\"type\":\"ConnectorPlacement.EquallySpacedConnector\",\"uuid\":\"6030dd83-63ea-4a67-9f73-95d000b3af89\"}],\"packageUris\":[\"http://schema.mathworks.com/mf0/Connector/R2020b\"],\"version\":\"1.0\"}"
  Terminator : Terminator
  Terminator2 : Terminator
  Voltage Measurement : spsVoltageMeasurementLib/Voltage Measurement  PhasorSimulation=off  OutputType=Complex  PSBequivalent=0
  Vsrc_high : spsDCVoltageSourceLib/DC Voltage Source  Amplitude=V_high  Measurements=None
  Vsrc_low : spsDCVoltageSourceLib/DC Voltage Source  Amplitude=V_low  Measurements=None
  Zero : Constant  Value=0  OutDataTypeStr=Inherit: Inherit via back propagation
  I_high : Outport
  I_low : Outport  Port=2
  VLf : Outport  Port=3
  P_h : Outport  Port=4
  wires:
  MOS_low/1 -> Terminator/1
  MOS_high/1 -> Terminator2/1
  [P_h] -> MOS_high/1
  [P_low] -> MOS_low/1
  Demux/1 -> I_high/1
  Demux/2 -> I_low/1, Control/2(Meas)
  [p] -> P_h/1, [P_h]
  i_ref/1 -> Control/1(Ref)
  Multimeter1/1 -> Abs/1
  Zero/1 -> [P_low]
  Abs/1 -> Demux/1
  Control/1(P) -> [p]
  Voltage Measurement/1 -> VLf/1
  connections:
  MOS_high/LConn1 -- Res_high/RConn1
  MOS_low/RConn1 -- Ground9/LConn1
  MOS_high/RConn1 -- MOS_low/LConn1 -- Voltage Measurement/LConn1 -- Ind_filt/LConn1 -- Subsystem1/LConn1
  Ground8/LConn1 -- Vsrc_high/LConn1
  Ground6/LConn1 -- Vsrc_low/LConn1
  Ind_filt/RConn1 -- Res_low/LConn1 -- Voltage Measurement/LConn2
  Res_high/LConn1 -- Vsrc_high/RConn1
  Res_low/RConn1 -- Vsrc_low/RConn1

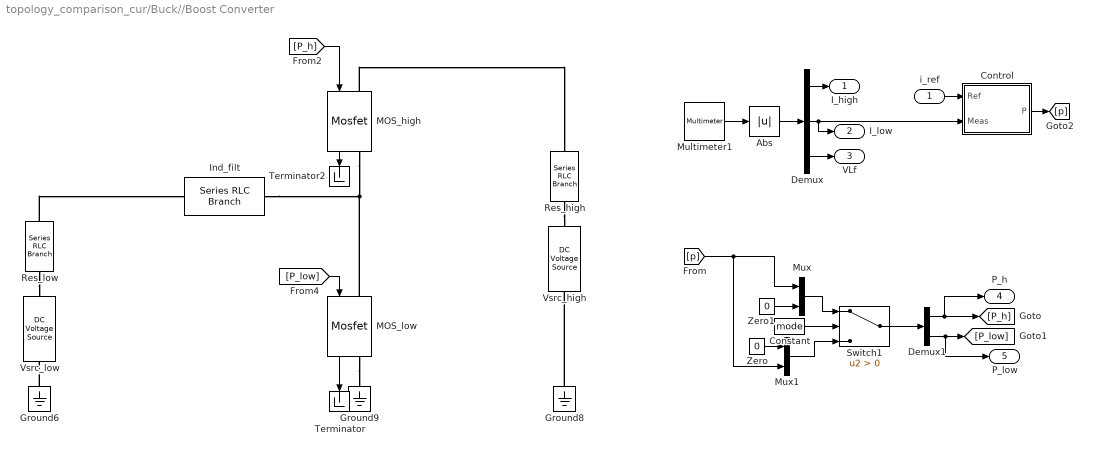
== system topology_comparison_cur/Buck//Boost Converter ==
  i_ref : Inport
  Abs : Abs  SaturateOnIntegerOverflow=off
  Constant : Constant  Value=mode
  Control : Subsystem
  Demux : Demux  Outputs=3
  Demux1 : Demux  Outputs=2
  Ground6 : spsGroundLib/Ground  LConnTagsString=a
  Ground8 : spsGroundLib/Ground  LConnTagsString=a
  Ground9 : spsGroundLib/Ground  LConnTagsString=a
  Ind_filt : spsSeriesRLCBranchLib/Series RLC Branch  LConnTagsString=__new0  RConnTagsString=__new0  BranchType=RL  Resistance=L_res  Inductance=L_ind*2  SetiL0=off  InitialCurrent=20  Capacitance=1e-6  Setx0=off  InitialVoltage=0  Measurements=Branch voltage
  MOS_high : spsMosfetLib/Mosfet  Ron=MOS_Ron  Lon=0  Rd=DIO_Ron  Vfd=MOS_Vfw  IC=0  Rs=1e5  Cs=inf  Measurements=on
  MOS_low : spsMosfetLib/Mosfet  Ron=MOS_Ron  Lon=0  Rd=DIO_Ron  Vfd=MOS_Vfw  IC=0  Rs=1e5  Cs=inf  Measurements=on
  Multimeter1 : spsMultimeterLib/Multimeter  L=12  sel=[7 8 1]  yselected={}  Gain=[1 1 1]  OutputType=Complex  PlotAtSimulationStop=off  PhasorSimulation=off
  Mux : Mux  Inputs=2
  Mux1 : Mux  Inputs=2
  Res_high : spsSeriesRLCBranchLib/Series RLC Branch  LConnTagsString=__new0  RConnTagsString=__new0  BranchType=R  Resistance=TRC_Res  Inductance=1e-3  SetiL0=off  InitialCurrent=0  Capacitance=1e-6  Setx0=off  InitialVoltage=0  Measurements=Branch current
  Res_low : spsSeriesRLCBranchLib/Series RLC Branch  LConnTagsString=__new0  RConnTagsString=__new0  BranchType=R  Resistance=TRC_Res  Inductance=1e-3  SetiL0=off  InitialCurrent=0  Capacitance=1e-6  Setx0=off  InitialVoltage=0  Measurements=Branch current
  Switch1 : Switch  Criteria=u2 > Threshold  SaturateOnIntegerOverflow=off  InputSameDT=off
  Terminator : Terminator
  Terminator2 : Terminator
  Vsrc_high : spsDCVoltageSourceLib/DC Voltage Source  Amplitude=V_high  Measurements=None
  Vsrc_low : spsDCVoltageSourceLib/DC Voltage Source  Amplitude=V_low  Measurements=None
  Zero : Constant  Value=0  OutDataTypeStr=Inherit: Inherit via back propagation
  Zero1 : Constant  Value=0  OutDataTypeStr=Inherit: Inherit via back propagation
  I_high : Outport
  I_low : Outport  Port=2
  VLf : Outport  Port=3
  P_h : Outport  Port=4
  P_low : Outport  Port=5
  wires:
  MOS_low/1 -> Terminator/1
  MOS_high/1 -> Terminator2/1
  [P_h] -> MOS_high/1
  [P_low] -> MOS_low/1
  Demux/1 -> I_high/1
  Demux/2 -> Control/2(Meas), I_low/1
  [p] -> Mux1/2, Mux/1
  Constant/1 -> Switch1/2
  Mux/1 -> Switch1/1
  Switch1/1 -> Demux1/1
  Demux1/1 -> P_h/1, [P_h]
  Zero/1 -> Mux1/1
  Mux1/1 -> Switch1/3
  i_ref/1 -> Control/1(Ref)
  Multimeter1/1 -> Abs/1
  Zero1/1 -> Mux/2
  Demux1/2 -> P_low/1, [P_low]
  Abs/1 -> Demux/1
  Control/1(P) -> [p]
  Demux/3 -> VLf/1
  connections:
  MOS_high/LConn1 -- Res_high/RConn1
  MOS_low/RConn1 -- Ground9/LConn1
  MOS_high/RConn1 -- Ind_filt/LConn1 -- MOS_low/LConn1
  Ground8/LConn1 -- Vsrc_high/LConn1
  Ground6/LConn1 -- Vsrc_low/LConn1
  Res_low/LConn1 -- Ind_filt/RConn1
  Res_high/LConn1 -- Vsrc_high/RConn1
  Res_low/RConn1 -- Vsrc_low/RConn1

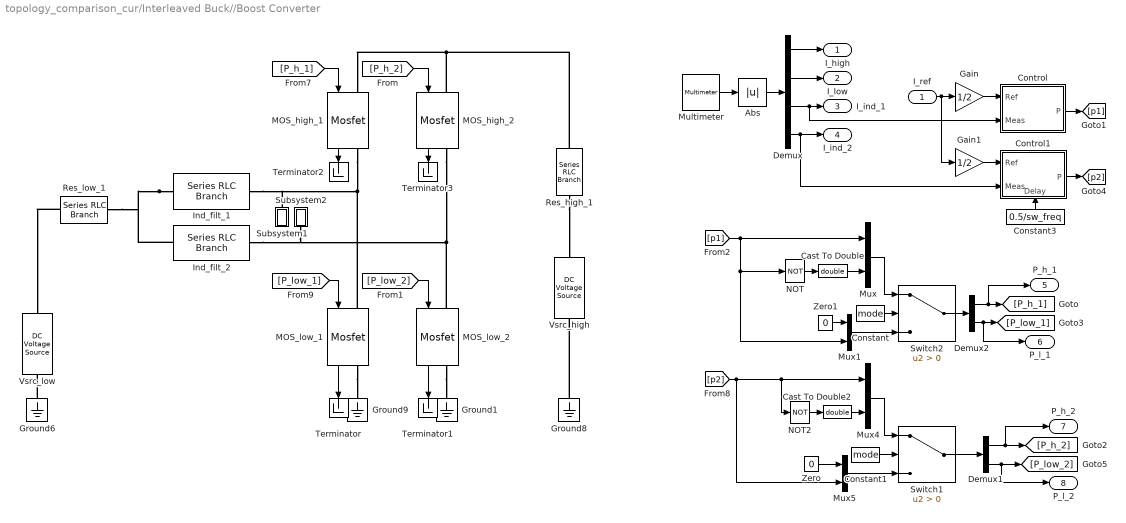
== system topology_comparison_cur/Interleaved Buck//Boost Converter ==
  I_ref : Inport
  Abs : Abs  SaturateOnIntegerOverflow=off
  Cast To Double : DataTypeConversion  OutDataTypeStr=double  SaturateOnIntegerOverflow=off  RndMeth=Floor
  Cast To Double2 : DataTypeConversion  OutDataTypeStr=double  SaturateOnIntegerOverflow=off  RndMeth=Floor
  Constant : Constant  Value=mode
  Constant1 : Constant  Value=mode
  Constant3 : Constant  Value=0.5/sw_freq
  Control : Subsystem
  Control1 : Subsystem
      settings: PortSchema="{\"entries\":[{\"content\":{\"sides\":[{\"content\":{\"connectorIds\":[\"In1\",\"In2\"]},\"type\":\"ConnectorPlacement.EquallySpacedRectSide\",\"uuid\":\"44975c06-6cb3-4b92-aa2e-c11b859d13e4\"},{\"content\":{\"connectorIds\":[\"Out1\"],\"side\":\"RIGHT\"},\"type\":\"ConnectorPlacement.EquallySpacedRectSide\",\"uuid\":\"ebdc9065-5b19-4aa7-8841-916fd82a5d31\"},{\"content\":{\"side\":\"TOP\"},\"type\":\"ConnectorPlacement.EquallySpacedRectSide\",\"uuid\":\"027925ea-888b-4bcf-b8a4-44694d0e275e\"},{\"content\":{\"connectorIds\":[\"In3\"],\"side\":\"BOTTOM\"},\"type\":\"ConnectorPlacement.EquallySpacedRectSide\",\"uuid\":\"4b21ce2f-6f21-43cd-b77f-3dbeff0cb919\"}]},\"type\":\"ConnectorPlacement.EquallySpacedConnector\",\"uuid\":\"3cd19595-535e-42c3-a0e6-40045bedee28\"}],\"packageUris\":[\"http://schema.mathworks.com/mf0/Connector/R2020b\"],\"version\":\"1.0\"}"
  Demux : Demux
  Demux1 : Demux  Outputs=2
  Demux2 : Demux  Outputs=2
  Gain : Gain  Gain=1/2
  Gain1 : Gain  Gain=1/2
  Ground{1,6,8..9} (4 alike) : spsGroundLib/Ground  LConnTagsString=a
  Ind_filt_1 : spsSeriesRLCBranchLib/Series RLC Branch  LConnTagsString=__new0  RConnTagsString=__new0  BranchType=RL  Resistance=L_res  Inductance=L_ind*10  SetiL0=off  InitialCurrent=10  Capacitance=1e-6  Setx0=off  InitialVoltage=0  Measurements=Branch current
  Ind_filt_2 : spsSeriesRLCBranchLib/Series RLC Branch  LConnTagsString=__new0  RConnTagsString=__new0  BranchType=RL  Resistance=L_res  Inductance=L_ind*10  SetiL0=off  InitialCurrent=10  Capacitance=1e-6  Setx0=off  InitialVoltage=0  Measurements=Branch current
  MOS_high_1 : spsMosfetLib/Mosfet  Ron=MOS_Ron  Lon=0  Rd=DIO_Ron  Vfd=MOS_Vfw  IC=0  Rs=1e5  Cs=inf  Measurements=on
  MOS_high_2 : spsMosfetLib/Mosfet  Ron=MOS_Ron  Lon=0  Rd=DIO_Ron  Vfd=MOS_Vfw  IC=0  Rs=1e5  Cs=inf  Measurements=on
  MOS_low_1 : spsMosfetLib/Mosfet  Ron=MOS_Ron  Lon=0  Rd=DIO_Ron  Vfd=MOS_Vfw  IC=0  Rs=1e5  Cs=inf  Measurements=on
  MOS_low_2 : spsMosfetLib/Mosfet  Ron=MOS_Ron  Lon=0  Rd=DIO_Ron  Vfd=MOS_Vfw  IC=0  Rs=1e5  Cs=inf  Measurements=on
  Multimeter : spsMultimeterLib/Multimeter  L=9  sel=[8 9 6 7]  yselected={}  Gain=[1 1 1 1]  OutputType=Complex  PlotAtSimulationStop=off  PhasorSimulation=off
  Mux{,1,4..5} (4 alike) : Mux  Inputs=2
  NOT : Logic  Operator=NOT  IconShape=distinctive  AllPortsSameDT=off  OutDataTypeStr=boolean
  NOT2 : Logic  Operator=NOT  IconShape=distinctive  AllPortsSameDT=off  OutDataTypeStr=boolean
  Res_high_1 : spsSeriesRLCBranchLib/Series RLC Branch  LConnTagsString=__new0  RConnTagsString=__new0  BranchType=R  Resistance=TRC_Res  Inductance=1e-3  SetiL0=off  InitialCurrent=0  Capacitance=1e-6  Setx0=off  InitialVoltage=0  Measurements=Branch current
  Res_low_1 : spsSeriesRLCBranchLib/Series RLC Branch  LConnTagsString=__new0  RConnTagsString=__new0  BranchType=R  Resistance=TRC_Res  Inductance=1e-3  SetiL0=off  InitialCurrent=0  Capacitance=1e-6  Setx0=off  InitialVoltage=0  Measurements=Branch current
  Subsystem1 : Subsystem
      settings: PortSchema="{\"entries\":[{\"content\":{\"sides\":[{\"content\":{},\"type\":\"ConnectorPlacement.EquallySpacedRectSide\",\"uuid\":\"333a472d-5660-403e-9749-9e5a485a4e51\"},{\"content\":{\"side\":\"RIGHT\"},\"type\":\"ConnectorPlacement.EquallySpacedRectSide\",\"uuid\":\"46e3a3df-9b43-4056-bf49-6d97e0ff375e\"},{\"content\":{\"connectorIds\":[\"LConn1\"],\"side\":\"TOP\"},\"type\":\"ConnectorPlacement.EquallySpacedRectSide\",\"uuid\":\"a9be43b9-3284-437d-b483-2a714199e3a2\"}]},\"type\":\"ConnectorPlacement.EquallySpacedConnector\",\"uuid\":\"6030dd83-63ea-4a67-9f73-95d000b3af89\"}],\"packageUris\":[\"http://schema.mathworks.com/mf0/Connector/R2020b\"],\"version\":\"1.0\"}"
  Subsystem2 : Subsystem
      settings: PortSchema="{\"entries\":[{\"content\":{\"sides\":[{\"content\":{},\"type\":\"ConnectorPlacement.EquallySpacedRectSide\",\"uuid\":\"333a472d-5660-403e-9749-9e5a485a4e51\"},{\"content\":{\"side\":\"RIGHT\"},\"type\":\"ConnectorPlacement.EquallySpacedRectSide\",\"uuid\":\"46e3a3df-9b43-4056-bf49-6d97e0ff375e\"},{\"content\":{\"connectorIds\":[\"LConn1\"],\"side\":\"TOP\"},\"type\":\"ConnectorPlacement.EquallySpacedRectSide\",\"uuid\":\"a9be43b9-3284-437d-b483-2a714199e3a2\"}]},\"type\":\"ConnectorPlacement.EquallySpacedConnector\",\"uuid\":\"6030dd83-63ea-4a67-9f73-95d000b3af89\"}],\"packageUris\":[\"http://schema.mathworks.com/mf0/Connector/R2020b\"],\"version\":\"1.0\"}"
  Switch1 : Switch  Criteria=u2 > Threshold  SaturateOnIntegerOverflow=off  InputSameDT=off
  Switch2 : Switch  Criteria=u2 > Threshold  SaturateOnIntegerOverflow=off  InputSameDT=off
  Terminator{,1..3} (4 alike) : Terminator
  Vsrc_high : spsDCVoltageSourceLib/DC Voltage Source  Amplitude=V_high  Measurements=None
  Vsrc_low : spsDCVoltageSourceLib/DC Voltage Source  Amplitude=V_low  Measurements=None
  Zero : Constant  Value=0  OutDataTypeStr=Inherit: Inherit via back propagation
  Zero1 : Constant  Value=0  OutDataTypeStr=Inherit: Inherit via back propagation
  I_high : Outport
  I_low : Outport  Port=2
  I_ind_1 : Outport  Port=3
  I_ind_2 : Outport  Port=4
  P_h_1 : Outport  Port=5
  P_l_1 : Outport  Port=6
  P_h_2 : Outport  Port=7
  P_l_2 : Outport  Port=8
  wires:
  [P_h_1] -> MOS_high_1/1
  [P_low_2] -> MOS_low_2/1
  MOS_high_1/1 -> Terminator2/1
  MOS_low_1/1 -> Terminator/1
  MOS_low_2/1 -> Terminator1/1
  MOS_high_2/1 -> Terminator3/1
  [P_low_1] -> MOS_low_1/1
  Multimeter/1 -> Abs/1
  Demux/3 -> Control/2(Meas), I_ind_1/1
  Constant/1 -> Switch2/2
  Demux2/2 -> P_l_1/1, [P_low_1]
  Mux/1 -> Switch2/1
  Mux1/1 -> Switch2/3
  Cast To Double/1 -> Mux/2
  [p1] -> Mux/1, NOT/1, Mux1/2
  [P_h_2] -> MOS_high_2/1
  Demux/2 -> I_low/1
  I_ref/1 -> Gain1/1, Gain/1
  Switch1/1 -> Demux1/1
  Demux1/1 -> P_h_2/1, [P_h_2]
  Switch2/1 -> Demux2/1
  Demux/1 -> I_high/1
  Abs/1 -> Demux/1
  Control/1(P) -> [p1]
  Gain/1 -> Control/1(Ref)
  Demux2/1 -> P_h_1/1, [P_h_1]
  Control1/1(P) -> [p2]
  Demux/4 -> Control1/2(Meas), I_ind_2/1
  Gain1/1 -> Control1/1(Ref)
  Constant1/1 -> Switch1/2
  Mux4/1 -> Switch1/1
  Mux5/1 -> Switch1/3
  Constant3/1 -> Control1/3(Delay)
  Demux1/2 -> P_l_2/1, [P_low_2]
  NOT/1 -> Cast To Double/1
  Zero1/1 -> Mux1/1
  NOT2/1 -> Cast To Double2/1
  Cast To Double2/1 -> Mux4/2
  [p2] -> NOT2/1, Mux4/1, Mux5/2
  Zero/1 -> Mux5/1
  connections:
  MOS_high_2/RConn1 -- Subsystem2/LConn1 -- Ind_filt_2/LConn1 -- MOS_low_2/LConn1
  MOS_high_1/RConn1 -- Ind_filt_1/LConn1 -- Subsystem1/LConn1 -- MOS_low_1/LConn1
  Ind_filt_1/RConn1 -- Ind_filt_2/RConn1 -- Res_low_1/LConn1
  Ground8/LConn1 -- Vsrc_high/LConn1
  MOS_low_1/RConn1 -- Ground9/LConn1
  Ground6/LConn1 -- Vsrc_low/LConn1
  MOS_low_2/RConn1 -- Ground1/LConn1
  Res_high_1/LConn1 -- Vsrc_high/RConn1
  Res_low_1/RConn1 -- Vsrc_low/RConn1
  Res_high_1/RConn1 -- MOS_high_2/LConn1 -- MOS_high_1/LConn1

== system topology_comparison_cur/Meas_Deal ==
  In : Inport
  Clock1 : Clock
  Switch1 : Switch  Criteria=u2 > Threshold  Threshold=meas_delay  SaturateOnIntegerOverflow=off  InputSameDT=off
  Zero1 : Constant  Value=0  OutDataTypeStr=Inherit: Inherit via back propagation
  Out : Outport
  wires:
  Zero1/1 -> Switch1/3
  Switch1/1 -> Out/1
  Clock1/1 -> Switch1/2
  In/1 -> Switch1/1

== system topology_comparison_cur/Meas_Deal1 ==
  In : Inport
  Clock1 : Clock
  Switch1 : Switch  Criteria=u2 > Threshold  Threshold=meas_delay  SaturateOnIntegerOverflow=off  InputSameDT=off
  Zero1 : Constant  Value=0  OutDataTypeStr=Inherit: Inherit via back propagation
  Out : Outport
  wires:
  Zero1/1 -> Switch1/3
  Switch1/1 -> Out/1
  Clock1/1 -> Switch1/2
  In/1 -> Switch1/1

== system topology_comparison_cur/Meas_Deal2 ==
  In : Inport
  Clock1 : Clock
  Switch1 : Switch  Criteria=u2 > Threshold  Threshold=meas_delay  SaturateOnIntegerOverflow=off  InputSameDT=off
  Zero1 : Constant  Value=0  OutDataTypeStr=Inherit: Inherit via back propagation
  Out : Outport
  wires:
  Zero1/1 -> Switch1/3
  Switch1/1 -> Out/1
  Clock1/1 -> Switch1/2
  In/1 -> Switch1/1

== system topology_comparison_cur/Meas_Deal3 ==
  In : Inport
  Clock1 : Clock
  Switch1 : Switch  Criteria=u2 > Threshold  Threshold=meas_delay  SaturateOnIntegerOverflow=off  InputSameDT=off
  Zero1 : Constant  Value=0  OutDataTypeStr=Inherit: Inherit via back propagation
  Out : Outport
  wires:
  Zero1/1 -> Switch1/3
  Switch1/1 -> Out/1
  Clock1/1 -> Switch1/2
  In/1 -> Switch1/1

== system topology_comparison_cur/Meas_Deal4 ==
  In : Inport
  Clock1 : Clock
  Switch1 : Switch  Criteria=u2 > Threshold  Threshold=meas_delay  SaturateOnIntegerOverflow=off  InputSameDT=off
  Zero1 : Constant  Value=0  OutDataTypeStr=Inherit: Inherit via back propagation
  Out : Outport
  wires:
  Zero1/1 -> Switch1/3
  Switch1/1 -> Out/1
  Clock1/1 -> Switch1/2
  In/1 -> Switch1/1

== system topology_comparison_cur/Meas_Deal5 ==
  In : Inport
  Clock1 : Clock
  Switch1 : Switch  Criteria=u2 > Threshold  Threshold=meas_delay  SaturateOnIntegerOverflow=off  InputSameDT=off
  Zero1 : Constant  Value=0  OutDataTypeStr=Inherit: Inherit via back propagation
  Out : Outport
  wires:
  Zero1/1 -> Switch1/3
  Switch1/1 -> Out/1
  Clock1/1 -> Switch1/2
  In/1 -> Switch1/1

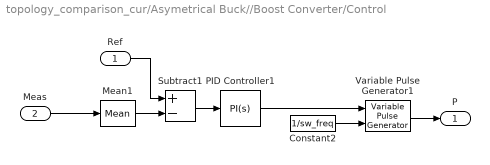
== system topology_comparison_cur/Asymetrical Buck//Boost Converter/Control ==
  Ref : Inport
  Meas : Inport  Port=2
  Constant2 : Constant  Value=1/sw_freq
  Mean1 : spsMeanLib/Mean  Freq=sw_freq/10  Vinit=0  Ts=0
  PID Controller1 : slpidlib/PID Controller  Controller=PI  Form=Parallel  TimeDomain=Continuous-time  UseExternalTs=off  SampleTime=-1  IntegratorMethod=Forward Euler  FilterMethod=Forward Euler  ControllerParametersSource=internal  P=asym_bdc_p  I=asym_bdc_i  UseKiTs=on  D=0  UseExternalDerivativeSource=off  N=100  UseFilter=on  TunerSelectOption=Transfer Function Based (PID Tuner App)  InitialConditionSource=internal  InitialConditionForIntegrator=0.15  InitialConditionForFilter=0.1  DifferentiatorICPrevScaledInput=0  ExternalReset=none  TrackingMode=off  Kt=1  LimitOutput=on  SatLimitsSource=internal  UpperSaturationLimit=1  LowerSaturationLimit=0.01  LinearizeAsGain=on  AntiWindupMode=none  Kb=1  LimitIntegrator=off  UpperIntegratorSaturationLimit=inf  LowerIntegratorSaturationLimit=-inf  POutMin=[]  POutMax=[]  IOutMin=[]  IOutMax=[]  DOutMin=[]  DOutMax=[]  NOutMin=[]  NOutMax=[]  SumOutMin=[]  SumOutMax=[]  SaturationOutMin=[]  SaturationOutMax=[]  PParamMin=[]  PParamMax=[]  IParamMin=[]  IParamMax=[]  DParamMin=[]  DParamMax=[]  NParamMin=[]  NParamMax=[]  KbParamMin=[]  KbParamMax=[]  KtParamMin=[]  KtParamMax=[]  KbOutMin=[]  KbOutMax=[]  KtOutMin=[]  KtOutMax=[]  IntegratorOutMin=[]  IntegratorOutMax=[]  FilterOutMin=[]  FilterOutMax=[]  SumI1OutMin=[]  SumI1OutMax=[]  SumI2OutMin=[]  SumI2OutMax=[]  SumI3OutMin=[]  SumI3OutMax=[]  SumI4OutMin=[]  SumI4OutMax=[]  SumDOutMin=[]  SumDOutMax=[]  DifferentiatorOutMin=[]  DifferentiatorOutMax=[]  FilterDiffOutCoefMin=[]  FilterDiffOutCoefMax=[]  ReciprocalOutMin=[]  ReciprocalOutMax=[]  SumDenOutMin=[]  SumDenOutMax=[]  SumNumOutMin=[]  SumNumOutMax=[]  DivideOutMin=[]  DivideOutMax=[]  UdiffTsProdOutMin=[]  UdiffTsProdOutMax=[]  NTsProdOutMin=[]  NTsProdOutMax=[]  UintegralTsProdOutMin=[]  UintegralTsProdOutMax=[]  UngainTsProdOutMin=[]  UngainTsProdOutMax=[]  ClampingZeroOutDataTypeStr=Inherit: Inherit via back propagation  ClampingZeroOutMin=[]  ClampingZeroOutMax=[]  FilterDenConstantOutDataTypeStr=Inherit: Inherit via back propagation  FilterDenConstantOutMin=[]  FilterDenConstantOutMax=[]  PCopyOutDataTypeStr=Inherit: Inherit via back propagation  PCopyOutMin=[]  PCopyOutMax=[]  NCopyOutDataTypeStr=Inherit: Inherit via back propagation  NCopyOutMin=[]  NCopyOutMax=[]  IntegratorContinuousStateAttributes=''  IntegratorStateMustResolveToSignalObject=off  IntegratorRTWStateStorageClass=Auto  FilterContinuousStateAttributes=''  FilterStateMustResolveToSignalObject=off  FilterRTWStateStorageClass=Auto  ParallelPVariant=InternalParameters  IdealPVariant=Disabled  IVariant=InternalParameters  DVariant=Disabled  IntegratorVariant=Continuous  SatVariant=Enabled  AWVariant=Passthrough  PCopyVariant=Disabled  TRVariant=Disabled  FdbkBlocksVariant=Forward  IdealPFdbkVariant=Disabled  SatFdbkVariant=Disabled  DerivativeFilterVariant=Disabled  NVariant=Disabled  NCopyVariant=Disabled_SignalSpec  FilterICVariant=Disabled  IntegratorICVariant=InternalICs  ExternalResetVariant=Disabled  TRSumVariant=Passthrough  SumFdbkVariant=Disabled  SumVariant=Sum_PI  TsampFilterVariant=InternalTs  TsampNgainVariant=Passthrough  TsampIntegralVariant=Disabled_SignalSpec  ExternalSaturationOutDataTypeStr=Inherit: Same as second input  DerivativeSourceVariant=Disabled  PreIntVariant=InternalPreInt
  Subtract1 : Sum  Inputs=+-
  Variable Pulse Generator1 : VariablePulseGenerator  AllowZeroPulseWidth=on  SampleTime=0.1
  P : Outport
  wires:
  Meas/1 -> Mean1/1
  PID Controller1/1 -> Variable Pulse Generator1/1
  Constant2/1 -> Variable Pulse Generator1/2
  Mean1/1 -> Subtract1/2
  Subtract1/1 -> PID Controller1/1
  Variable Pulse Generator1/1 -> P/1
  Ref/1 -> Subtract1/1
